simulink model "bloc simulink"  (R2014a)
settings: Solver=ode45  StartTime=0.0  StopTime=10.0  RelTol=1e-3
settings Model: Creator=ARSINE  LastModifiedBy=ARSINE

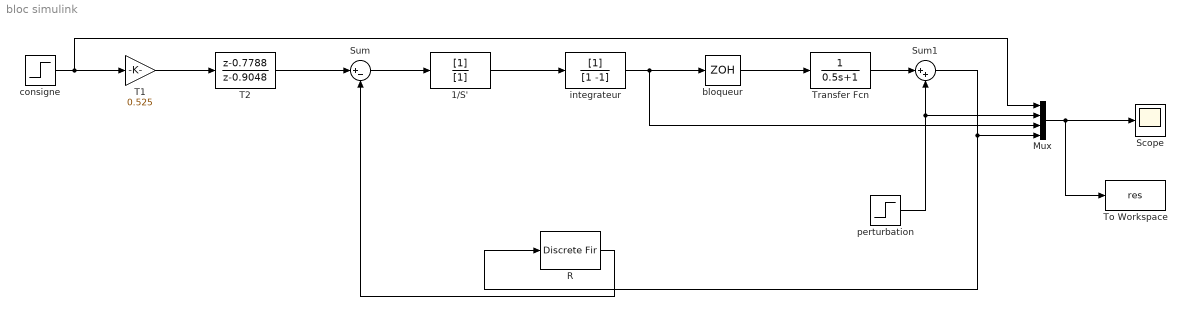
== system bloc simulink ==
  "1/S' " : DiscreteFilter  Denominator=[1]  SampleTime=0.1
  Mux : Mux
  "R  " : DiscreteFir  Coefficients=[5.7369 -4.5166]  SampleTime=0.1
  Scope : Scope
  Sum : Sum  Inputs=|+-  SampleTime=0.1
  Sum1 : Sum  Inputs=|++
  T1 : Gain  Gain=0.525  SampleTime=0.1
  "T2 " : DiscreteTransferFcn  Numerator=[1 -0.7788]  Denominator=[1 -0.9048]  SampleTime=0.1
  To Workspace : ToWorkspace  VariableName=res  SaveFormat=Timeseries  SampleTime=-1
  Transfer Fcn : TransferFcn  Denominator=[0.5 1]
  "bloqueur " : ZeroOrderHold  SampleTime=0.1
  consigne : Step  Time=0  After=0.3  SampleTime=0.1
  "integrateur " : DiscreteFilter  Denominator=[1 -1]  SampleTime=0.1
  perturbation : Step  Time=2  After=0.05  SampleTime=0.1
  wires:
  T1/1 -> "T2 "/1
  "T2 "/1 -> Sum/1
  Sum/1 -> "1/S' "/1
  "1/S' "/1 -> "integrateur "/1
  "integrateur "/1 -> Mux/3, "bloqueur "/1
  "bloqueur "/1 -> Transfer Fcn/1
  Transfer Fcn/1 -> Sum1/1
  Sum1/1 -> "R  "/1, Mux/4
  "R  "/1 -> Sum/2
  consigne/1 -> T1/1, Mux/1
  perturbation/1 -> Mux/2, Sum1/2
  Mux/1 -> Scope/1, To Workspace/1
